simulink model "pondera"  (R2020b)
settings: Solver=VariableStepAuto  StartTime=0.0  StopTime=20  RelTol=1e-3
settings Model: Creator=diosdado  LastModifiedBy=diosdado

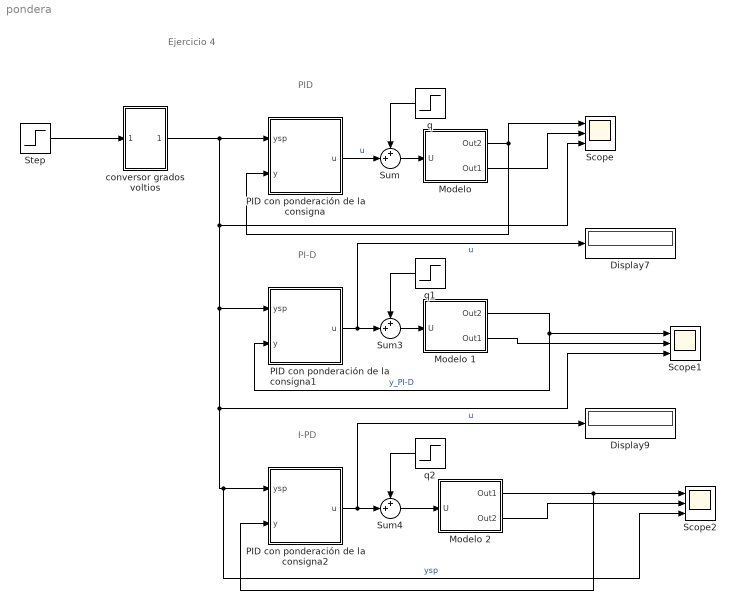
== system pondera ==
  note: Ejercicio 4
  note: PID
  note: PI-D
  note: I-PD
  Display7 : Display
  Display9 : Display
  "Modelo " : Subsystem
  Modelo 1 : Subsystem
  Modelo 2 : Subsystem
  PID con ponderación de la consigna : Subsystem  mask{Kp=100/40, Ti=1.17/1.96, Td=0.118/1.17, b=0, c=0, N=30}
      mask prompts: Kp "Ganancia Proporcional (Kp)"; Ti "Tiempo Integral (Ti) [s]"; Td "Tiempo Derivativo (Td) [s]"; b "Peso Error Proporcional (b)"; c "Peso Error Derivativo (c)"; N "Filtro Derivativo (N) [rad/s]"
  PID con ponderación de la consigna1 : Subsystem  mask{Kp=2.5, Ti=1.17/1.96, Td=0.118/1.17, b=0, c=0, N=30}
      mask prompts: Kp "Ganancia Proporcional (Kp)"; Ti "Tiempo Integral (Ti) [s]"; Td "Tiempo Derivativo (Td) [s]"; b "Peso Error Proporcional (b)"; c "Peso Error Derivativo (c)"; N "Filtro Derivativo (N) [rad/s]"
  PID con ponderación de la consigna2 : Subsystem  mask{Kp=100/40, Ti=1.17/1.96, Td=0.118/1.17, b=0, c=0, N=30}
      mask prompts: Kp "Ganancia Proporcional (Kp)"; Ti "Tiempo Integral (Ti) [s]"; Td "Tiempo Derivativo (Td) [s]"; b "Peso Error Proporcional (b)"; c "Peso Error Derivativo (c)"; N "Filtro Derivativo (N) [rad/s]"
  Scope : Scope  NumInputPorts=3
  Scope1 : Scope  NumInputPorts=3
  Scope2 : Scope  NumInputPorts=3
  Step : Step  Before=10  After=30  SampleTime=0
  Sum : Sum  Inputs=++|
  Sum3 : Sum  Inputs=++|
  Sum4 : Sum  Inputs=++|
  "conversor grados voltios " : Subsystem  mask{a=4.95, b=0.869}
  q : Step  Time=15  After=0.5  SampleTime=0
  q1 : Step  Time=15  After=0.5  SampleTime=0
  q2 : Step  Time=15  After=0.5  SampleTime=0
  wires:
  q/1 -> Sum/1
  "conversor grados voltios "/1(Out1) -> PID con ponderación de la consigna/1(ysp), Scope/3, Scope1/3, Scope2/3, PID con ponderación de la consigna2/1(ysp), PID con ponderación de la consigna1/1(ysp)  "ysp"
  Sum3/1 -> Modelo 1/1(U)
  PID con ponderación de la consigna/1(u) -> Sum/2  "u"
  Sum/1 -> "Modelo "/1(U)
  PID con ponderación de la consigna1/1(u) -> Sum3/2, Display7/1  "u"
  q1/1 -> Sum3/1
  Modelo 1/1(Out2) -> PID con ponderación de la consigna1/2(y), Scope1/1  "y_PI-D"
  Sum4/1 -> Modelo 2/1(U)
  PID con ponderación de la consigna2/1(u) -> Sum4/2, Display9/1  "u"
  q2/1 -> Sum4/1
  "Modelo "/1(Out2) -> Scope/1, PID con ponderación de la consigna/2(y)
  "Modelo "/2(Out1) -> Scope/2
  Modelo 1/2(Out1) -> Scope1/2
  Modelo 2/1(Out1) -> PID con ponderación de la consigna2/2(y), Scope2/1
  Modelo 2/2(Out2) -> Scope2/2
  Step/1 -> "conversor grados voltios "/1(In1)

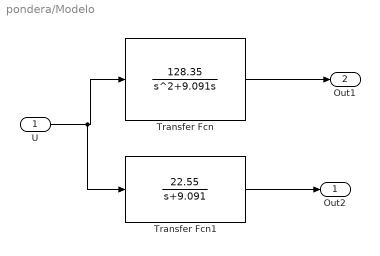
== system pondera/Modelo  ==
  U : Inport
  Transfer Fcn : TransferFcn  Numerator=[128.35]  Denominator=[1 9.091 0]
  Transfer Fcn1 : TransferFcn  Numerator=[22.55]  Denominator=[1 9.091]
  Out2 : Outport
  Out1 : Outport  Port=2
  wires:
  U/1 -> Transfer Fcn1/1, Transfer Fcn/1
  Transfer Fcn/1 -> Out1/1
  Transfer Fcn1/1 -> Out2/1

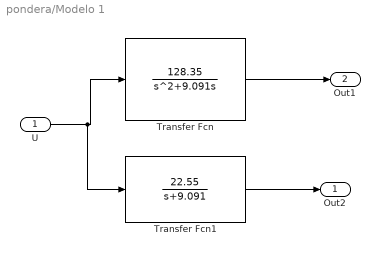
== system pondera/Modelo 1 ==
  U : Inport
  Transfer Fcn : TransferFcn  Numerator=[128.35]  Denominator=[1 9.091 0]
  Transfer Fcn1 : TransferFcn  Numerator=[22.55]  Denominator=[1 9.091]
  Out2 : Outport
  Out1 : Outport  Port=2
  wires:
  U/1 -> Transfer Fcn1/1, Transfer Fcn/1
  Transfer Fcn/1 -> Out1/1
  Transfer Fcn1/1 -> Out2/1

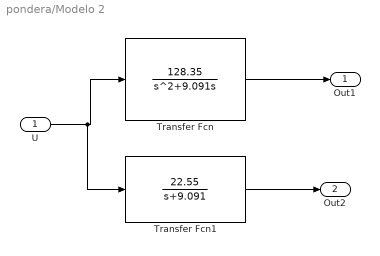
== system pondera/Modelo 2 ==
  U : Inport
  Transfer Fcn : TransferFcn  Numerator=[128.35]  Denominator=[1 9.091 0]
  Transfer Fcn1 : TransferFcn  Numerator=[22.55]  Denominator=[1 9.091]
  Out1 : Outport
  Out2 : Outport  Port=2
  wires:
  U/1 -> Transfer Fcn1/1, Transfer Fcn/1
  Transfer Fcn/1 -> Out1/1
  Transfer Fcn1/1 -> Out2/1

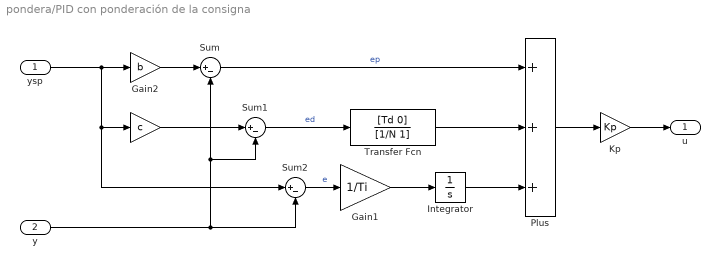
== system pondera/PID con ponderación de la consigna ==
  ysp : Inport
  y : Inport  Port=2
  " " : Gain  Gain=c
  Gain1 : Gain  Gain=1/Ti
  Gain2 : Gain  Gain=b
  Integrator : Integrator
  Kp : Gain  Gain=Kp
  Plus : Sum  Inputs=+++
  Sum : Sum  Inputs=|+-
  Sum1 : Sum  Inputs=|+-
  Sum2 : Sum  Inputs=|+-
  Transfer Fcn : TransferFcn  Numerator=[Td 0]  Denominator=[1/N 1]
  u : Outport  VectorParamsAs1DForOutWhenUnconnected=off
  wires:
  Plus/1 -> Kp/1
  Kp/1 -> u/1
  Gain1/1 -> Integrator/1
  Integrator/1 -> Plus/3
  Transfer Fcn/1 -> Plus/2
  ysp/1 -> Sum2/1, " "/1, Gain2/1
  Gain2/1 -> Sum/1
  Sum/1 -> Plus/1  "ep"
  " "/1 -> Sum1/1
  Sum2/1 -> Gain1/1  "e"
  Sum1/1 -> Transfer Fcn/1  "ed"
  y/1 -> Sum/2, Sum1/2, Sum2/2

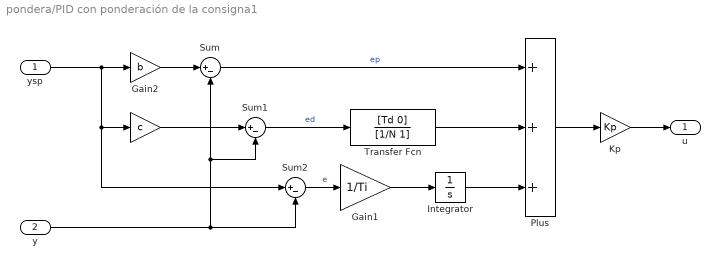
== system pondera/PID con ponderación de la consigna1 ==
  ysp : Inport
  y : Inport  Port=2
  " " : Gain  Gain=c
  Gain1 : Gain  Gain=1/Ti
  Gain2 : Gain  Gain=b
  Integrator : Integrator
  Kp : Gain  Gain=Kp
  Plus : Sum  Inputs=+++
  Sum : Sum  Inputs=|+-
  Sum1 : Sum  Inputs=|+-
  Sum2 : Sum  Inputs=|+-
  Transfer Fcn : TransferFcn  Numerator=[Td 0]  Denominator=[1/N 1]
  u : Outport  VectorParamsAs1DForOutWhenUnconnected=off
  wires:
  Plus/1 -> Kp/1
  Kp/1 -> u/1
  Gain1/1 -> Integrator/1
  Integrator/1 -> Plus/3
  Transfer Fcn/1 -> Plus/2
  ysp/1 -> Sum2/1, " "/1, Gain2/1
  Gain2/1 -> Sum/1
  Sum/1 -> Plus/1  "ep"
  " "/1 -> Sum1/1
  Sum2/1 -> Gain1/1  "e"
  Sum1/1 -> Transfer Fcn/1  "ed"
  y/1 -> Sum/2, Sum1/2, Sum2/2

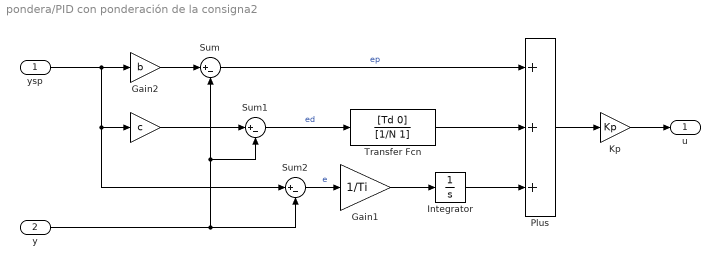
== system pondera/PID con ponderación de la consigna2 ==
  ysp : Inport
  y : Inport  Port=2
  " " : Gain  Gain=c
  Gain1 : Gain  Gain=1/Ti
  Gain2 : Gain  Gain=b
  Integrator : Integrator
  Kp : Gain  Gain=Kp
  Plus : Sum  Inputs=+++
  Sum : Sum  Inputs=|+-
  Sum1 : Sum  Inputs=|+-
  Sum2 : Sum  Inputs=|+-
  Transfer Fcn : TransferFcn  Numerator=[Td 0]  Denominator=[1/N 1]
  u : Outport  VectorParamsAs1DForOutWhenUnconnected=off
  wires:
  Plus/1 -> Kp/1
  Kp/1 -> u/1
  Gain1/1 -> Integrator/1
  Integrator/1 -> Plus/3
  Transfer Fcn/1 -> Plus/2
  ysp/1 -> Sum2/1, " "/1, Gain2/1
  Gain2/1 -> Sum/1
  Sum/1 -> Plus/1  "ep"
  " "/1 -> Sum1/1
  Sum2/1 -> Gain1/1  "e"
  Sum1/1 -> Transfer Fcn/1  "ed"
  y/1 -> Sum/2, Sum1/2, Sum2/2

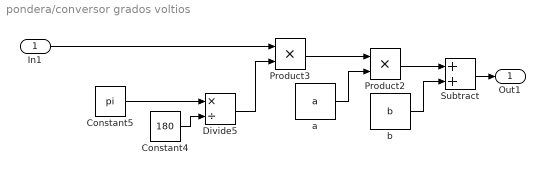
== system pondera/conversor grados voltios  ==
  In1 : Inport
  Constant4 : Constant  Value=180
  Constant5 : Constant  Value=pi
  Divide5 : Product  Inputs=*/
  Product2 : Product
  Product3 : Product
  Subtract : Sum
  a : Constant  Value=a
  b : Constant  Value=b
  Out1 : Outport
  wires:
  b/1 -> Subtract/2
  Product3/1 -> Product2/1
  Constant4/1 -> Divide5/2
  In1/1 -> Product3/1
  Product2/1 -> Subtract/1
  a/1 -> Product2/2
  Constant5/1 -> Divide5/1
  Divide5/1 -> Product3/2
  Subtract/1 -> Out1/1
